simulink model "LongCtrl_14"  (R2019b)
settings: Solver=VariableStepAuto  StartTime=0.0  StopTime=10.0  RelTol=1e-3
libraries: simulink x9, simulink_extras x1
settings Model: Creator=ED1  LastModifiedBy=ED1

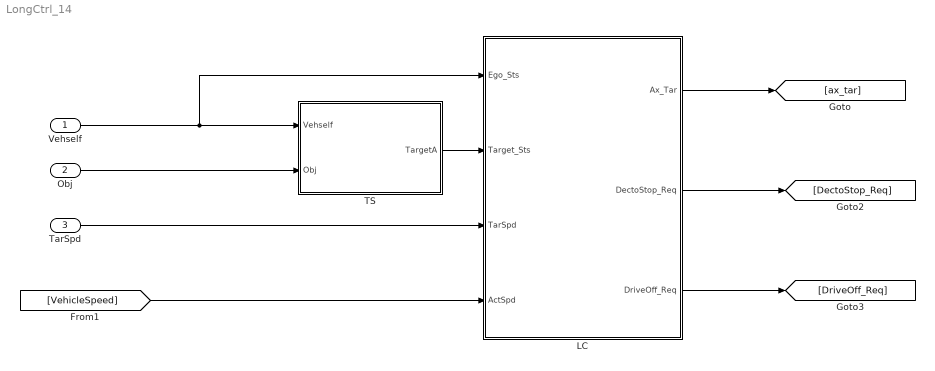
== system LongCtrl_14 ==
  Vehself : Inport  OutDataTypeStr=Bus:VehSelf1Vcc
  Obj : Inport  Port=2  OutDataTypeStr=Bus:ObjGroup1Vcc  PortDimensions=32  BusOutputAsStruct=on
  TarSpd : Inport  Port=3
  LC : Subsystem
  TS : Subsystem
  wires:
  TarSpd/1 -> LC/3(TarSpd)
  LC/2(DectoStop_Req) -> [DectoStop_Req]
  LC/3(DriveOff_Req) -> [DriveOff_Req]
  LC/1(Ax_Tar) -> [ax_tar]
  Obj/1 -> TS/2(Obj)
  [VehicleSpeed] -> LC/4(ActSpd)
  Vehself/1 -> LC/1(Ego_Sts), TS/1(Vehself)
  TS/1(TargetA) -> LC/2(Target_Sts)

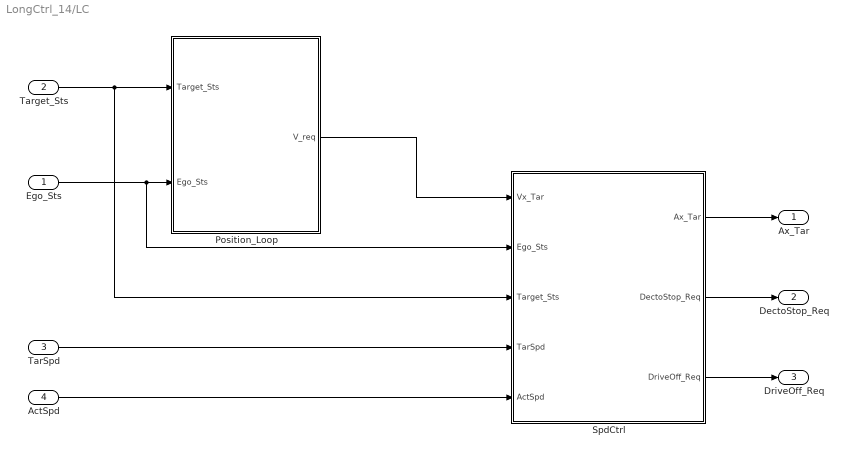
== system LongCtrl_14/LC ==
  Ego_Sts : Inport
  Target_Sts : Inport  Port=2
  TarSpd : Inport  Port=3
  ActSpd : Inport  Port=4
  Position_Loop : Subsystem
  SpdCtrl : Subsystem
  Ax_Tar : Outport
  DectoStop_Req : Outport  Port=2
  DriveOff_Req : Outport  Port=3
  wires:
  Ego_Sts/1 -> Position_Loop/2(Ego_Sts), SpdCtrl/2(Ego_Sts)
  SpdCtrl/2(DectoStop_Req) -> DectoStop_Req/1
  TarSpd/1 -> SpdCtrl/4(TarSpd)
  Position_Loop/1(V_req) -> SpdCtrl/1(Vx_Tar)
  Target_Sts/1 -> Position_Loop/1(Target_Sts), SpdCtrl/3(Target_Sts)
  SpdCtrl/3(DriveOff_Req) -> DriveOff_Req/1
  SpdCtrl/1(Ax_Tar) -> Ax_Tar/1
  ActSpd/1 -> SpdCtrl/5(ActSpd)

== system LongCtrl_14/TS ==
  Vehself : Inport  OutDataTypeStr=Bus:VehSelf1Vcc
  Obj : Inport  Port=2  OutDataTypeStr=Bus:ObjGroup1Vcc
  TargetSelection : MATLAB Function  TreatAsAtomicUnit=on
  TargetA : Outport  OutDataTypeStr=Bus: TargetADZJ
  wires:
  Obj/1 -> TargetSelection/2(objects)
  Vehself/1 -> TargetSelection/1(vehself)
  TargetSelection/1(TargetA) -> TargetA/1

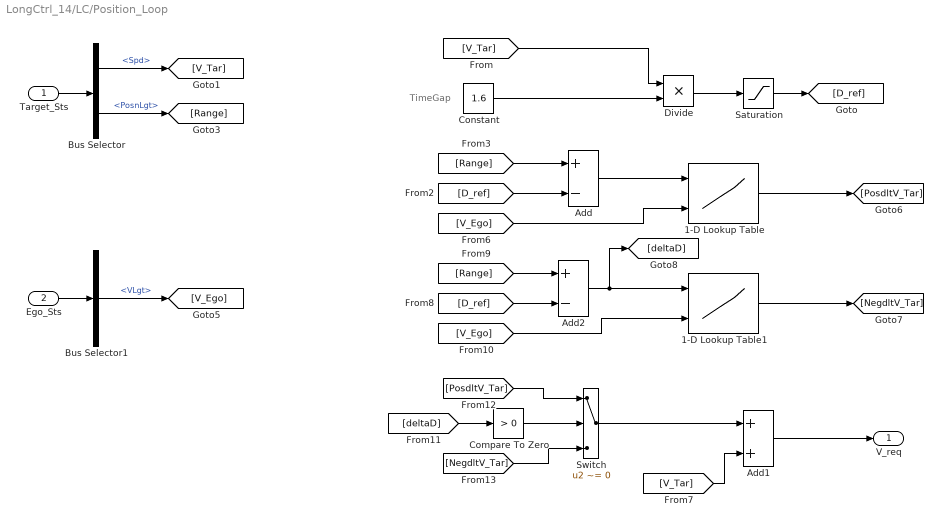
== system LongCtrl_14/LC/Position_Loop ==
  note: TimeGap
  Target_Sts : Inport
  Ego_Sts : Inport  Port=2
  1-D Lookup Table : Lookup_n-D  BreakpointsForDimension1=single([0,5,10,20,40,60,80,100]);  BreakpointsForDimension2=single([0,8.300000190734863]);  Table=single(reshape([0,1,1.2,1.8,2.5,2.5,2.5,2.5,0,1,1.2,1.8,3,3,3,3],8,2));  ExtrapMethod=Clip  UseLastTableValue=on  InternalRulePriority=Speed  RndMeth=Simplest  InputSameDT=on
  1-D Lookup Table1 : Lookup_n-D  BreakpointsForDimension1=single([-7 -5 0])  BreakpointsForDimension2=single([0 8.3])  Table=single([-0.7 -0.7 0;-1.2 -1.2 0]')  ExtrapMethod=Clip  UseLastTableValue=on  InternalRulePriority=Speed  RndMeth=Simplest  InputSameDT=on
  Add : Sum  Inputs=+-
  Add1 : Sum
  Add2 : Sum  Inputs=+-
  Bus Selector : BusSelector  OutputSignals=Spd,PosnLgt
  Bus Selector1 : BusSelector  OutputSignals=VLgt
  Compare To Zero : simulink/Logic and Bit Operations/Compare To Zero  relop=>  OutDataTypeStr=boolean
  Constant : Constant  Value=1.6  OutDataTypeStr=single
  Divide : Product  Inputs=**
  Saturation : Saturate  UpperLimit=100  LowerLimit=5
  Switch : Switch  Criteria=u2 ~= 0
  V_req : Outport
  wires:
  Saturation/1 -> [D_ref]
  [NegdltV_Tar] -> Switch/3
  [D_ref] -> Add2/2
  [Range] -> Add2/1
  [PosdltV_Tar] -> Switch/1
  [deltaD] -> Compare To Zero/1
  Switch/1 -> Add1/1
  Compare To Zero/1 -> Switch/2
  Add2/1 -> 1-D Lookup Table1/1, [deltaD]
  [V_Ego] -> 1-D Lookup Table1/2
  1-D Lookup Table1/1 -> [NegdltV_Tar]
  Add1/1 -> V_req/1
  [V_Tar] -> Add1/2
  1-D Lookup Table/1 -> [PosdltV_Tar]
  [V_Ego] -> 1-D Lookup Table/2
  [Range] -> Add/1
  Add/1 -> 1-D Lookup Table/1
  [D_ref] -> Add/2
  Divide/1 -> Saturation/1
  Constant/1 -> Divide/2
  [V_Tar] -> Divide/1
  Bus Selector1/1 -> [V_Ego]  "<VLgt>"
  Ego_Sts/1 -> Bus Selector1/1
  Bus Selector/2 -> [Range]  "<PosnLgt>"
  Bus Selector/1 -> [V_Tar]  "<Spd>"
  Target_Sts/1 -> Bus Selector/1

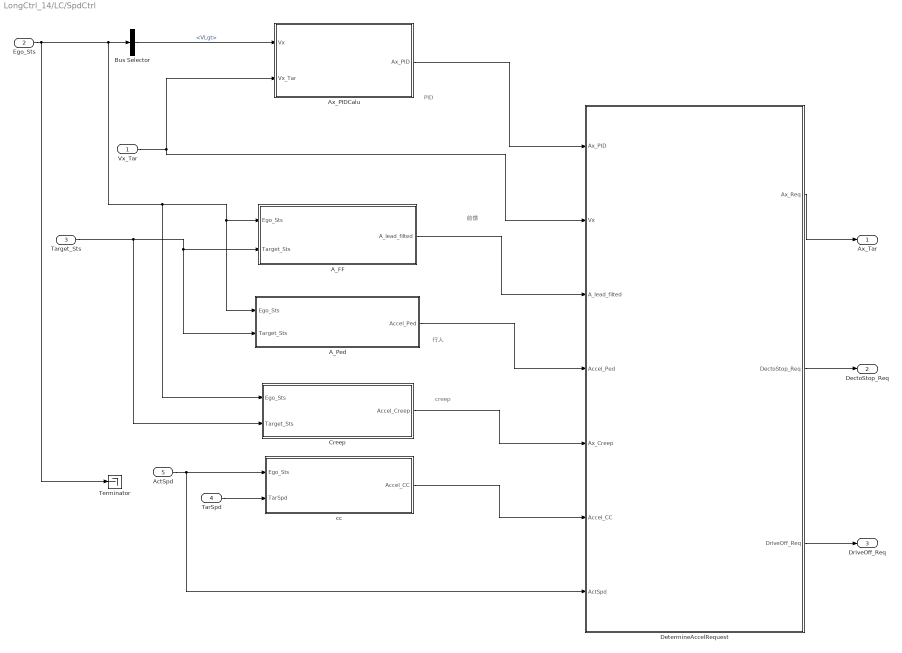
== system LongCtrl_14/LC/SpdCtrl ==
  note: 前馈
  note: PID
  note: 行人
  note: creep
  Vx_Tar : Inport  OutDataTypeStr=single
  Ego_Sts : Inport  Port=2
  Target_Sts : Inport  Port=3
  TarSpd : Inport  Port=4
  ActSpd : Inport  Port=5
  A_FF : Subsystem
  A_Ped : Subsystem
  Ax_PIDCalu : Subsystem
  Bus Selector : BusSelector  OutputSignals=VLgt
  Creep : Subsystem
  DetermineAccelRequest : Subsystem
  Terminator : Terminator
  cc : Subsystem
  Ax_Tar : Outport
  DectoStop_Req : Outport  Port=2
  DriveOff_Req : Outport  Port=3
  wires:
  Creep/1(Accel_Creep) -> DetermineAccelRequest/5(Ax_Creep)
  Ego_Sts/1 -> Terminator/1, A_Ped/1(Ego_Sts), A_FF/1(Ego_Sts), Creep/1(Ego_Sts), Bus Selector/1
  A_Ped/1(Accel_Ped) -> DetermineAccelRequest/4(Accel_Ped)
  A_FF/1(A_lead_filted) -> DetermineAccelRequest/3(A_lead_filted)
  Target_Sts/1 -> A_FF/2(Target_Sts), A_Ped/2(Target_Sts), Creep/2(Target_Sts)
  DetermineAccelRequest/1(Ax_Req) -> Ax_Tar/1
  Vx_Tar/1 -> Ax_PIDCalu/2(Vx_Tar), DetermineAccelRequest/2(Vx)
  Ax_PIDCalu/1(Ax_PID) -> DetermineAccelRequest/1(Ax_PID)
  Bus Selector/1 -> Ax_PIDCalu/1(Vx)  "<VLgt>"
  TarSpd/1 -> cc/2(TarSpd)
  cc/1(Accel_CC) -> DetermineAccelRequest/6(Accel_CC)
  ActSpd/1 -> DetermineAccelRequest/7(ActSpd), cc/1(Ego_Sts)
  DetermineAccelRequest/2(DectoStop_Req) -> DectoStop_Req/1
  DetermineAccelRequest/3(DriveOff_Req) -> DriveOff_Req/1

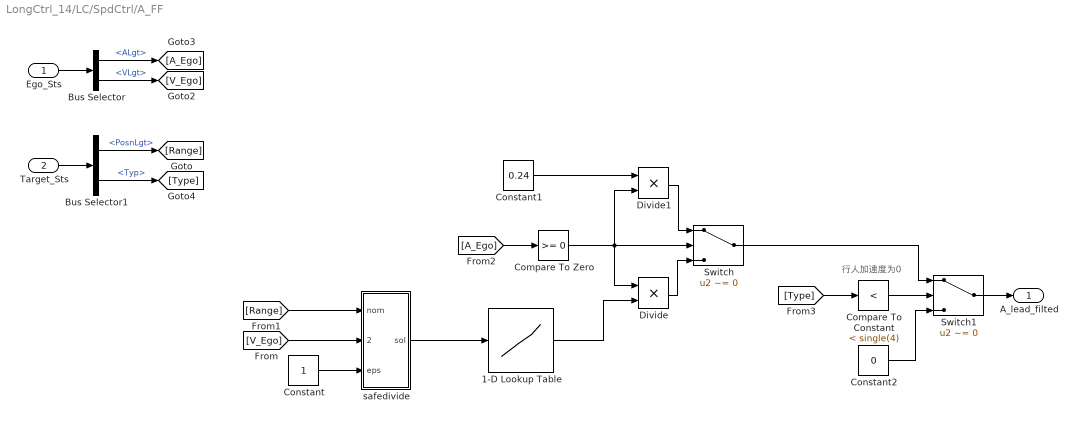
== system LongCtrl_14/LC/SpdCtrl/A_FF ==
  note: 行人加速度为0
  Ego_Sts : Inport
  Target_Sts : Inport  Port=2
  1-D Lookup Table : Lookup_n-D  NumberOfTableDimensions=1  BreakpointsForDimension1=single([0 0.8 4])  Table=single([1.6 0.93 0])  InternalRulePriority=Speed  RndMeth=Simplest  InputSameDT=on
  Bus Selector : BusSelector  OutputSignals=ALgt,VLgt
  Bus Selector1 : BusSelector  OutputSignals=PosnLgt,Typ
  Compare To Constant : simulink/Logic and Bit Operations/Compare To Constant  relop=<  const=single(4)  OutDataTypeStr=boolean
  Compare To Zero : simulink/Logic and Bit Operations/Compare To Zero  relop=>=  OutDataTypeStr=boolean
  Constant : Constant  OutDataTypeStr=single
  Constant1 : Constant  Value=0.24  OutDataTypeStr=single
  Constant2 : Constant  Value=0  OutDataTypeStr=single
  Divide : Product  Inputs=**
  Divide1 : Product  Inputs=**
  Switch : Switch  Criteria=u2 ~= 0
  Switch1 : Switch  Criteria=u2 ~= 0
  safedivide : Subsystem
  A_lead_filted : Outport
  wires:
  Constant2/1 -> Switch1/3
  Switch1/1 -> A_lead_filted/1
  Compare To Constant/1 -> Switch1/2
  [Type] -> Compare To Constant/1
  Bus Selector1/2 -> [Type]  "<Typ>"
  Constant1/1 -> Divide1/1
  Divide1/1 -> Switch/1
  Divide/1 -> Switch/3
  Compare To Zero/1 -> Switch/2, Divide/1, Divide1/2
  Switch/1 -> Switch1/1
  1-D Lookup Table/1 -> Divide/2
  [A_Ego] -> Compare To Zero/1
  safedivide/1(sol) -> 1-D Lookup Table/1
  Constant/1 -> safedivide/3(eps)
  [Range] -> safedivide/1(nom)
  [V_Ego] -> safedivide/2(denom)
  Bus Selector1/1 -> [Range]  "<PosnLgt>"
  Bus Selector/2 -> [V_Ego]  "<VLgt>"
  Target_Sts/1 -> Bus Selector1/1
  Bus Selector/1 -> [A_Ego]  "<ALgt>"
  Ego_Sts/1 -> Bus Selector/1

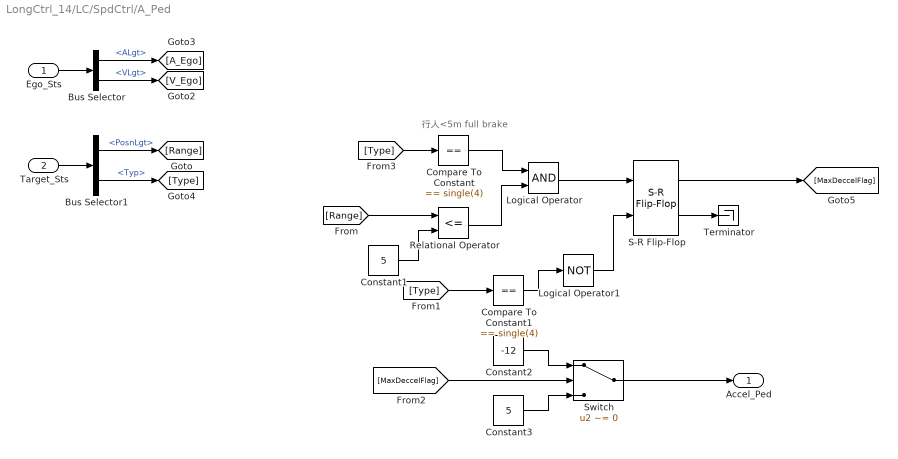
== system LongCtrl_14/LC/SpdCtrl/A_Ped ==
  note: 行人<5m full brake
  Ego_Sts : Inport
  Target_Sts : Inport  Port=2
  Bus Selector : BusSelector  OutputSignals=ALgt,VLgt
  Bus Selector1 : BusSelector  OutputSignals=PosnLgt,Typ
  Compare To Constant : simulink/Logic and Bit Operations/Compare To Constant  relop===  const=single(4)  OutDataTypeStr=boolean
  Compare To Constant1 : simulink/Logic and Bit Operations/Compare To Constant  relop===  const=single(4)  OutDataTypeStr=boolean
  Constant1 : Constant  Value=5  OutDataTypeStr=single
  Constant2 : Constant  Value=-12  OutDataTypeStr=single
  Constant3 : Constant  Value=5  OutDataTypeStr=single
  Logical Operator : Logic  AllPortsSameDT=off  OutDataTypeStr=boolean
  Logical Operator1 : Logic  Operator=NOT  AllPortsSameDT=off  OutDataTypeStr=boolean
  Relational Operator : RelationalOperator  Operator=<=  OutDataTypeStr=boolean  RndMeth=Simplest
  S-R Flip-Flop : simulink_extras/Flip Flops/S-R Flip-Flop  initial_condition=0
  Switch : Switch  Criteria=u2 ~= 0
  Terminator : Terminator
  Accel_Ped : Outport
  wires:
  Switch/1 -> Accel_Ped/1
  Constant3/1 -> Switch/3
  Constant2/1 -> Switch/1
  [MaxDeccelFlag] -> Switch/2
  S-R Flip-Flop/1 -> [MaxDeccelFlag]
  Logical Operator1/1 -> S-R Flip-Flop/2
  Compare To Constant1/1 -> Logical Operator1/1
  [Type] -> Compare To Constant1/1
  Constant1/1 -> Relational Operator/2
  [Range] -> Relational Operator/1
  S-R Flip-Flop/2 -> Terminator/1
  Relational Operator/1 -> Logical Operator/2
  Compare To Constant/1 -> Logical Operator/1
  Logical Operator/1 -> S-R Flip-Flop/1
  [Type] -> Compare To Constant/1
  Ego_Sts/1 -> Bus Selector/1
  Bus Selector/1 -> [A_Ego]  "<ALgt>"
  Target_Sts/1 -> Bus Selector1/1
  Bus Selector/2 -> [V_Ego]  "<VLgt>"
  Bus Selector1/1 -> [Range]  "<PosnLgt>"
  Bus Selector1/2 -> [Type]  "<Typ>"

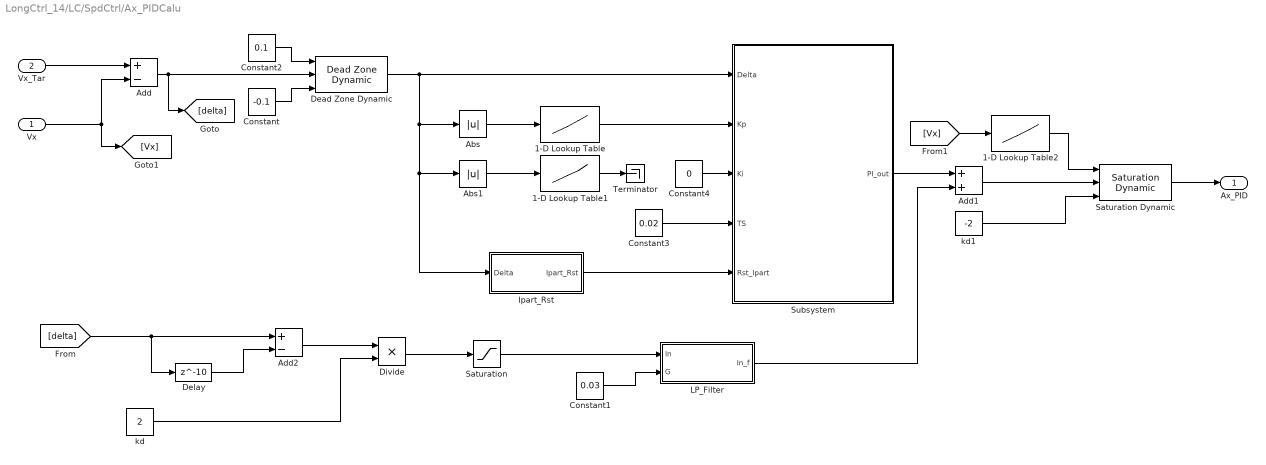
== system LongCtrl_14/LC/SpdCtrl/Ax_PIDCalu ==
  Vx : Inport
  Vx_Tar : Inport  Port=2
  1-D Lookup Table : Lookup_n-D  NumberOfTableDimensions=1  BreakpointsForDimension1=[0 1 2 3 4 5]  Table=[0.4 0.6 1.0 1.8 2 2]  ExtrapMethod=Clip  UseLastTableValue=on  InternalRulePriority=Speed  RndMeth=Simplest  InputSameDT=on
  1-D Lookup Table1 : Lookup_n-D  NumberOfTableDimensions=1  BreakpointsForDimension1=[0 2 5]  Table=[0.1 0.2 0.4]  ExtrapMethod=Clip  UseLastTableValue=on  InternalRulePriority=Speed  RndMeth=Simplest  InputSameDT=on
  1-D Lookup Table2 : Lookup_n-D  NumberOfTableDimensions=1  BreakpointsForDimension1=[0 15]  Table=[2 1.7]  ExtrapMethod=Clip  UseLastTableValue=on  InternalRulePriority=Speed  RndMeth=Simplest  InputSameDT=on
  Abs : Abs
  Abs1 : Abs
  Add : Sum  Inputs=+-
  Add1 : Sum
  Add2 : Sum  Inputs=+-
  Constant : Constant  Value=-0.1  OutDataTypeStr=single
  Constant1 : Constant  Value=0.03  OutDataTypeStr=single
  Constant2 : Constant  Value=0.1  OutDataTypeStr=single
  Constant3 : Constant  Value=0.02  OutDataTypeStr=single
  Constant4 : Constant  Value=0  OutDataTypeStr=single
  Dead Zone Dynamic : simulink/Discontinuities/Dead Zone Dynamic
      settings: SourceProductName=Simulink  SourceProductBaseCode=SL
  Delay : Delay  DelayLength=10  InitialCondition=0
  Divide : Product  Inputs=**
  Ipart_Rst : Subsystem
  LP_Filter : Subsystem
  Saturation : Saturate
  Saturation Dynamic : simulink/Discontinuities/Saturation Dynamic  OutMin=[]  OutMax=[]  OutDataTypeStr=Inherit: Same as second input  OutDataType=fixdt(1, 16)  OutScaling=2^-10  DoSatur=off
  Subsystem : Subsystem
  Terminator : Terminator
  kd : Constant  Value=2  OutDataTypeStr=single
  kd1 : Constant  Value=-2  OutDataTypeStr=single
  Ax_PID : Outport
  wires:
  kd1/1 -> Saturation Dynamic/3
  [Vx] -> 1-D Lookup Table2/1
  1-D Lookup Table2/1 -> Saturation Dynamic/1
  Saturation Dynamic/1 -> Ax_PID/1
  Constant4/1 -> Subsystem/3(Ki)
  Subsystem/1(PI_out) -> Add1/1
  Add/1 -> Dead Zone Dynamic/2, [delta]
  Constant3/1 -> Subsystem/4(TS)
  Saturation/1 -> LP_Filter/1(In)
  kd/1 -> Divide/2
  1-D Lookup Table/1 -> Subsystem/2(Kp)
  Constant/1 -> Dead Zone Dynamic/3
  [delta] -> Add2/1, Delay/1
  Delay/1 -> Add2/2
  Abs1/1 -> 1-D Lookup Table1/1
  Vx/1 -> [Vx], Add/2
  Vx_Tar/1 -> Add/1
  Add2/1 -> Divide/1
  Constant1/1 -> LP_Filter/2(G)
  Constant2/1 -> Dead Zone Dynamic/1
  Abs/1 -> 1-D Lookup Table/1
  LP_Filter/1(In_f) -> Add1/2
  1-D Lookup Table1/1 -> Terminator/1
  Add1/1 -> Saturation Dynamic/2
  Ipart_Rst/1(Ipart_Rst) -> Subsystem/5(Rst_Ipart)
  Divide/1 -> Saturation/1
  Dead Zone Dynamic/1 -> Subsystem/1(Delta), Ipart_Rst/1(Delta), Abs1/1, Abs/1

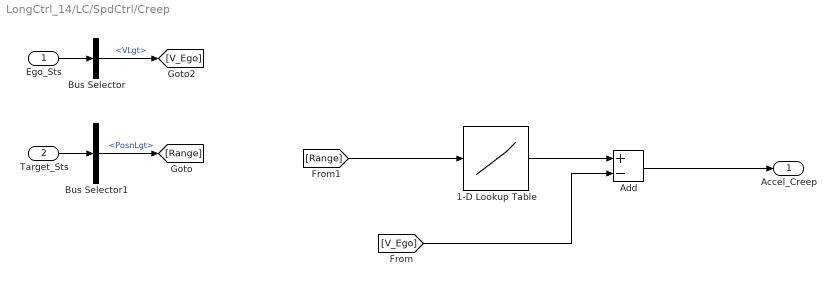
== system LongCtrl_14/LC/SpdCtrl/Creep ==
  Ego_Sts : Inport
  Target_Sts : Inport  Port=2
  1-D Lookup Table : Lookup_n-D  NumberOfTableDimensions=1  BreakpointsForDimension1=[2.5 3 4 6 7 11 16 26]  Table=[-5 -1 0 0.5 0.7 1.1 2 4]  InternalRulePriority=Speed  RndMeth=Simplest  InputSameDT=on
  Add : Sum  Inputs=+-
  Bus Selector : BusSelector  OutputSignals=VLgt
  Bus Selector1 : BusSelector  OutputSignals=PosnLgt
  Accel_Creep : Outport
  wires:
  [Range] -> 1-D Lookup Table/1
  [V_Ego] -> Add/2
  1-D Lookup Table/1 -> Add/1
  Add/1 -> Accel_Creep/1
  Bus Selector1/1 -> [Range]  "<PosnLgt>"
  Bus Selector/1 -> [V_Ego]  "<VLgt>"
  Target_Sts/1 -> Bus Selector1/1
  Ego_Sts/1 -> Bus Selector/1

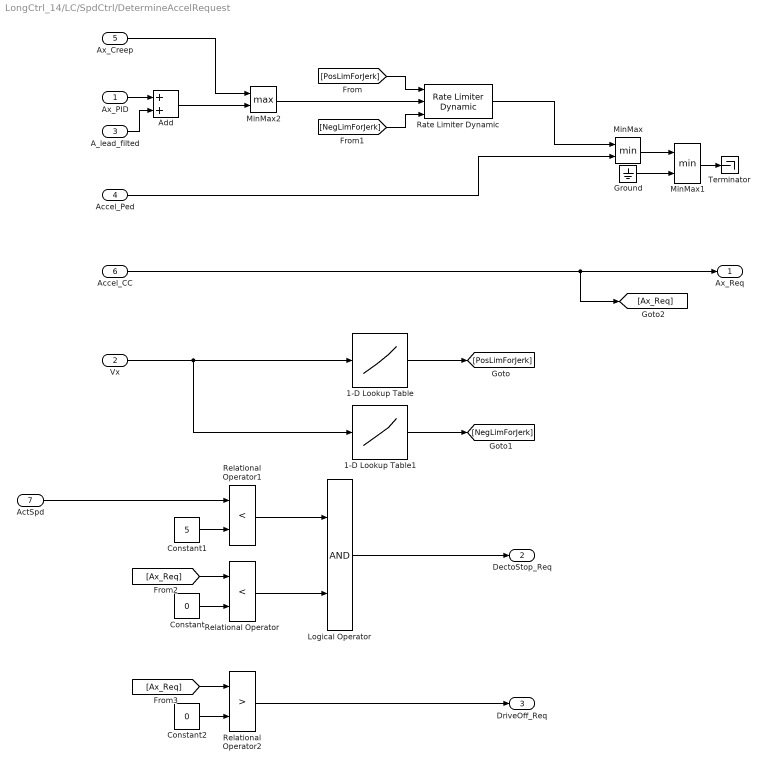
== system LongCtrl_14/LC/SpdCtrl/DetermineAccelRequest ==
  Ax_PID : Inport
  Vx : Inport  Port=2
  A_lead_filted : Inport  Port=3
  Accel_Ped : Inport  Port=4
  Ax_Creep : Inport  Port=5
  Accel_CC : Inport  Port=6
  ActSpd : Inport  Port=7
  1-D Lookup Table : Lookup_n-D  NumberOfTableDimensions=1  BreakpointsForDimension1=single([0 15 40 80 100 120 160 200]/3.6)  Table=single([2 1.5 1 1 1 1 1 1 ])  InternalRulePriority=Speed  RndMeth=Simplest  InputSameDT=on
  1-D Lookup Table1 : Lookup_n-D  NumberOfTableDimensions=1  BreakpointsForDimension1=single([0 15 40 80 100 120 160 200]/3.6)  Table=single([2 1.5 1 1 1 1 1 1 ]*-1)  InternalRulePriority=Speed  RndMeth=Simplest  InputSameDT=on
  Add : Sum
  Constant : Constant  Value=0
  Constant1 : Constant  Value=5
  Constant2 : Constant  Value=0
  Ground : Ground
  Logical Operator : Logic  AllPortsSameDT=off  OutDataTypeStr=boolean
  MinMax : MinMax  Inputs=2
  MinMax1 : MinMax  Inputs=2
  MinMax2 : MinMax  Function=max  Inputs=2
  Rate Limiter Dynamic : simulink/Discontinuities/Rate Limiter Dynamic
      settings: SourceProductName=Simulink
  Relational Operator : RelationalOperator  Operator=<  OutDataTypeStr=boolean  RndMeth=Simplest
  Relational Operator1 : RelationalOperator  Operator=<  OutDataTypeStr=boolean  RndMeth=Simplest
  Relational Operator2 : RelationalOperator  Operator=>  OutDataTypeStr=boolean  RndMeth=Simplest
  Terminator : Terminator
  Ax_Req : Outport
  DectoStop_Req : Outport  Port=2
  DriveOff_Req : Outport  Port=3
  wires:
  Add/1 -> MinMax2/2
  Ax_Creep/1 -> MinMax2/1
  Accel_Ped/1 -> MinMax/2
  A_lead_filted/1 -> Add/2
  Ax_PID/1 -> Add/1
  Rate Limiter Dynamic/1 -> MinMax/1
  1-D Lookup Table1/1 -> [NegLimForJerk]
  1-D Lookup Table/1 -> [PosLimForJerk]
  Vx/1 -> 1-D Lookup Table1/1, 1-D Lookup Table/1
  [NegLimForJerk] -> Rate Limiter Dynamic/3
  MinMax2/1 -> Rate Limiter Dynamic/2
  [PosLimForJerk] -> Rate Limiter Dynamic/1
  Accel_CC/1 -> [Ax_Req], Ax_Req/1
  MinMax/1 -> MinMax1/1
  Ground/1 -> MinMax1/2
  MinMax1/1 -> Terminator/1
  Constant/1 -> Relational Operator/2
  Relational Operator/1 -> Logical Operator/2
  ActSpd/1 -> Relational Operator1/1
  Constant1/1 -> Relational Operator1/2
  Relational Operator1/1 -> Logical Operator/1
  Logical Operator/1 -> DectoStop_Req/1
  [Ax_Req] -> Relational Operator/1
  [Ax_Req] -> Relational Operator2/1
  Constant2/1 -> Relational Operator2/2
  Relational Operator2/1 -> DriveOff_Req/1

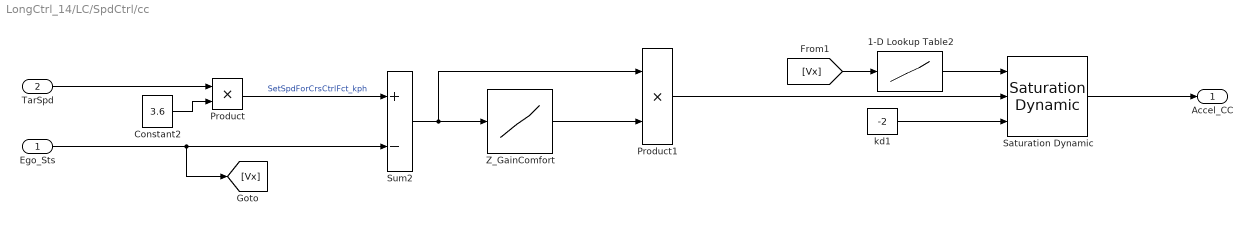
== system LongCtrl_14/LC/SpdCtrl/cc ==
  Ego_Sts : Inport
  TarSpd : Inport  Port=2
  1-D Lookup Table2 : Lookup_n-D  NumberOfTableDimensions=1  BreakpointsForDimension1=[0 15]  Table=[2 1.7]  ExtrapMethod=Clip  UseLastTableValue=on  InternalRulePriority=Speed  RndMeth=Simplest  InputSameDT=on
  Constant2 : Constant  Value=3.6  OutDataTypeStr=single
  Product : Product  RndMeth=Zero
  Product1 : Product  RndMeth=Zero
  Saturation Dynamic : simulink/Discontinuities/Saturation Dynamic  OutMin=[]  OutMax=[]  OutDataTypeStr=Inherit: Same as second input  OutDataType=fixdt(1, 16)  OutScaling=2^-10  DoSatur=off
  Sum2 : Sum  Tag=struct('comment',struct('text','','placement',1),'logdata',struct('maxnumvals',4096,'plotchannels',[],'stepsize',0,'downsampling',1,'loggingmode',3,'channels',1),'output',struct('width',1,'name','$S_$B','unit','','type','Float32','offset',0,'max',NaN,'min',NaN,'freeze',1,'lsb',1,'arb',0,'class','default','address','','description','','autoscalingmode',1,'lowerheadroom',1,'upperheadroom',1,'headroomunit','bit','checkmin',0,'checkmax',0,'show',0),'inputs','-+','date',731279.670781944)  Description=|  Inputs=+-  OutMin=-20  OutMax=20
      | Sum block of dSPACE TargetLink.
      | 
      | Output signal is equal to the sum of the input signals.
      | The list of signs is specified according to conventions for Simulink Sum blocks.
  Z_GainComfort : Lookup_n-D  NumberOfTableDimensions=1  BreakpointsForDimension1=single([ -10 -3 -1 3 10 ])  BreakpointsForDimension1DataTypeStr=Inherit: Inherit from 'Breakpoint data'  Table=single([ 0.1 0.1 0.075 0.075 0.075 ])  TableDataTypeStr=Inherit: Inherit from 'Table data'  OutDataTypeStr=Inherit: Inherit from 'Table data'  RndMeth=Simplest
  kd1 : Constant  Value=-2  OutDataTypeStr=single
  Accel_CC : Outport
  wires:
  Product/1 -> Sum2/1  "SetSpdForCrsCtrlFct_kph"
  Constant2/1 -> Product/2
  TarSpd/1 -> Product/1
  Sum2/1 -> Product1/1, Z_GainComfort/1
  Z_GainComfort/1 -> Product1/2
  kd1/1 -> Saturation Dynamic/3
  1-D Lookup Table2/1 -> Saturation Dynamic/1
  [Vx] -> 1-D Lookup Table2/1
  Saturation Dynamic/1 -> Accel_CC/1
  Product1/1 -> Saturation Dynamic/2
  Ego_Sts/1 -> [Vx], Sum2/2

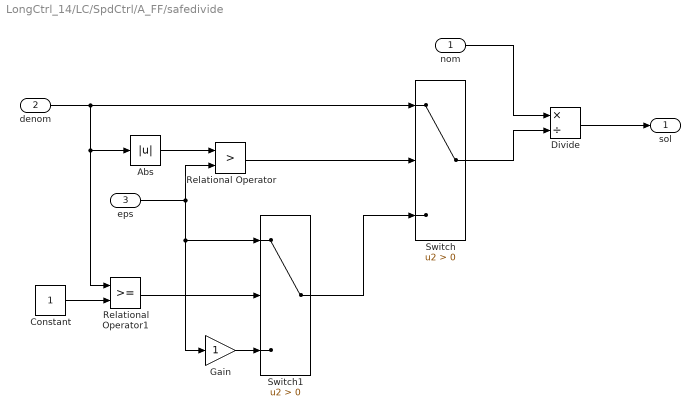
== system LongCtrl_14/LC/SpdCtrl/A_FF/safedivide ==
  nom : Inport
  denom : Inport  Port=2
  eps : Inport  Port=3
  Abs : Abs
  Constant : Constant  OutDataTypeStr=single
  Divide : Product  Inputs=*/
  Gain : Gain  ParamDataTypeStr=single
  Relational Operator : RelationalOperator  Operator=>  OutDataTypeStr=boolean  RndMeth=Simplest
  Relational Operator1 : RelationalOperator  OutDataTypeStr=boolean  RndMeth=Simplest
  Switch : Switch  Criteria=u2 > Threshold
  Switch1 : Switch  Criteria=u2 > Threshold
  sol : Outport
  wires:
  Divide/1 -> sol/1
  nom/1 -> Divide/1
  Switch/1 -> Divide/2
  Switch1/1 -> Switch/3
  Gain/1 -> Switch1/3
  Constant/1 -> Relational Operator1/2
  Relational Operator1/1 -> Switch1/2
  Relational Operator/1 -> Switch/2
  denom/1 -> Switch/1, Abs/1, Relational Operator1/1
  Abs/1 -> Relational Operator/1
  eps/1 -> Relational Operator/2, Gain/1, Switch1/1

== system LongCtrl_14/LC/SpdCtrl/Ax_PIDCalu/Ipart_Rst ==
  Delta : Inport
  Delay : Delay  DelayLength=1  InitialCondition=0
  Logical Operator : Logic  Operator=NOT  AllPortsSameDT=off  OutDataTypeStr=boolean
  Relational Operator : RelationalOperator  Operator===  OutDataTypeStr=boolean  RndMeth=Simplest
  Sign : Signum
  Ipart_Rst : Outport
  wires:
  Delay/1 -> Relational Operator/2
  Sign/1 -> Relational Operator/1, Delay/1
  Logical Operator/1 -> Ipart_Rst/1
  Relational Operator/1 -> Logical Operator/1
  Delta/1 -> Sign/1

== system LongCtrl_14/LC/SpdCtrl/Ax_PIDCalu/LP_Filter ==
  In : Inport
  G : Inport  Port=2
  Add : Sum  Inputs=-+
  Add1 : Sum
  Delay : Delay  DelayLength=1  InitialCondition=0
  Divide : Product  Inputs=**
  Divide1 : Product  Inputs=**
  In_f : Outport
  wires:
  Delay/1 -> Add/2, Divide1/2
  Add1/1 -> In_f/1, Delay/1
  Add/1 -> Add1/2
  Divide/1 -> Add1/1
  Divide1/1 -> Add/1
  G/1 -> Divide1/1, Divide/2
  In/1 -> Divide/1

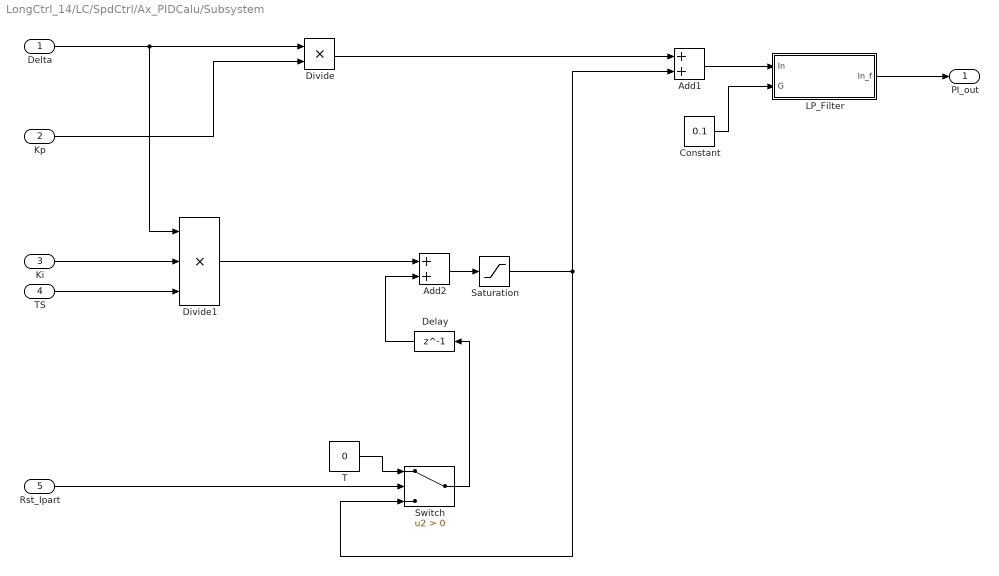
== system LongCtrl_14/LC/SpdCtrl/Ax_PIDCalu/Subsystem ==
  Delta : Inport
  Kp : Inport  Port=2
  Ki : Inport  Port=3
  TS : Inport  Port=4
  Rst_Ipart : Inport  Port=5
  Add1 : Sum
  Add2 : Sum
  Constant : Constant  Value=0.1  OutDataTypeStr=single
  Delay : Delay  DelayLength=1  InitialCondition=0
  Divide : Product  Inputs=**
  Divide1 : Product  Inputs=***
  LP_Filter : Subsystem
  Saturation : Saturate
  Switch : Switch  Criteria=u2 > Threshold
  T : Constant  Value=0  OutDataTypeStr=single
  PI_out : Outport
  wires:
  LP_Filter/1(In_f) -> PI_out/1
  Constant/1 -> LP_Filter/2(G)
  Add1/1 -> LP_Filter/1(In)
  Add2/1 -> Saturation/1
  Saturation/1 -> Switch/3, Add1/2
  Divide/1 -> Add1/1
  Switch/1 -> Delay/1
  T/1 -> Switch/1
  Rst_Ipart/1 -> Switch/2
  Delay/1 -> Add2/2
  Divide1/1 -> Add2/1
  Ki/1 -> Divide1/2
  TS/1 -> Divide1/3
  Kp/1 -> Divide/2
  Delta/1 -> Divide/1, Divide1/1

== system LongCtrl_14/LC/SpdCtrl/Ax_PIDCalu/Subsystem/LP_Filter ==
  In : Inport
  G : Inport  Port=2
  Add : Sum  Inputs=-+
  Add1 : Sum
  Delay : Delay  DelayLength=1  InitialCondition=0
  Divide : Product  Inputs=**
  Divide1 : Product  Inputs=**
  In_f : Outport
  wires:
  Delay/1 -> Add/2, Divide1/2
  Add1/1 -> In_f/1, Delay/1
  Add/1 -> Add1/2
  Divide/1 -> Add1/1
  Divide1/1 -> Add/1
  G/1 -> Divide1/1, Divide/2
  In/1 -> Divide/1

== matlab function LongCtrl_14/TS/TargetSelection ==
  data: vehself input; objects input; TargetA output Bus: TargetADZJ =0
function TargetA = fcn(vehself,objects)

TargetA = createAccATarget(vehself,objects);

end



function target = createAccATarget(vehself,objects)

    cip = getcip(objects);
    target = coder.nullcopy(struct( ...
        'Idn', uint8(0), ...
        'Spd', single(0), ...
        'PosnLgt', single(0), ...
        'ALgt', single(0), ...
        'Typ', uint8(0)));
          
    if cip > 0
        target.Idn = objects(cip).Ppty.Idn;
        target.Spd = objects(cip).Estimn.VLgt;
        target.PosnLgt = objects(cip).Estimn.PosnLgt;
        target.ALgt = objects(cip).Estimn.ALgt;
        target.Typ = uint8(objects(cip).Info.Typ);
    else
        target.Idn = cast(0, class(target.Idn));
        target.Spd = cast(vehself.VLgt, class(target.Spd));
        target.PosnLgt = cast(255, class(target.PosnLgt));
        target.ALgt = cast(0, class(target.ALgt));
        target.Typ = cast(0, class(target.Typ));
    end
end

function id = getcip(objects)
         id = 0;
         maxValue = single(200);
for i=1:32
     if abs(objects(i).Estimn.PosnLat) <= single(1.5)
         if objects(i).Estimn.PosnLgt < maxValue
             maxValue = objects(i).Estimn.PosnLgt;
             id = i;
         end
     end
end  
end
